simulink model "tester37311"  (R2022b)
settings: Solver=VariableStepAuto  StartTime=0.0  StopTime=25  RelTol=1e-3
values from neighbouring files (symbols this model uses):
  IPR = 0.99    [dane.m]    (also in tester23.m; wykresownik33.m; wykresownik35.m; wykresownik36.m)
  Ng_safe = 1.25    [dane.m]    (also in tester23.m; wykresownik33.m; wykresownik35.m; wykresownik36.m)
  Np = linspace(0.5,2,101)    [dane.m]    (also in tester23.m; untitled.m = 2303; wykresownik33.m; wykresownik35.m)
  Np_safe = 1.25    [dane.m]    (also in tester23.m; wykresownik33.m; wykresownik35.m; wykresownik36.m)
  optimal_rotation = 11.8694    [dane.m]    (also in wykresownik37311.m; wykresownikfinalny.m)
  P3tDIVP2t_perf = 1.0101    [dane.m]    (also in tester23.m = 1; wykresownik33.m = 1; wykresownik35.m = 1; wykresownik36.m = 1)
  P3tDIVP2t_safe = 1.35    [dane.m]    (also in tester23.m; wykresownik33.m; wykresownik35.m; wykresownik36.m)
  Q = 1./Np    [dane.m]    (also in tester23.m; wykresownik33.m; wykresownik35.m; wykresownik36.m)
  Q_safe = 1.15    [dane.m]    (also in tester23.m; wykresownik33.m; wykresownik35.m; wykresownik36.m)
  T45_perf = 1    [dane.m]    (also in tester23.m; wykresownik33.m; wykresownik35.m; wykresownik36.m)
  T45_safe = 1.3    [dane.m]    (also in tester23.m; wykresownik33.m; wykresownik35.m; wykresownik36.m)
  Wf = max(min((1-xfuel)*44,55),33)/1000    [dane.m]    (also in wykresownik37311.m; wykresownikfinalny.m = max(min((1-xfuel)*44,55),33)/100)
  xfuel = linspace(-1,1,201)    [dane.m]    (also in wykresownik37311.m; wykresownikfinalny.m)
libraries: fl_lib x5, sh_lib x4, nesl_utility x4, slpidlib x2, simulink x1
settings Model: Creator=48519  LastModifiedBy=48519
settings ModelReferenceCC: EnableRefExpFcnMdlSchedulingChecks=on

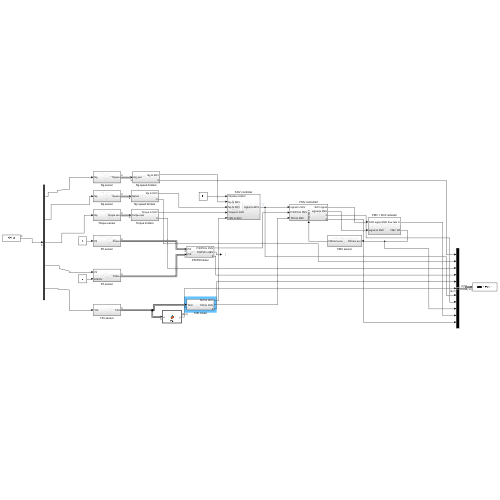
[thumbnail: Simulink's stored preview of the top-level diagram]
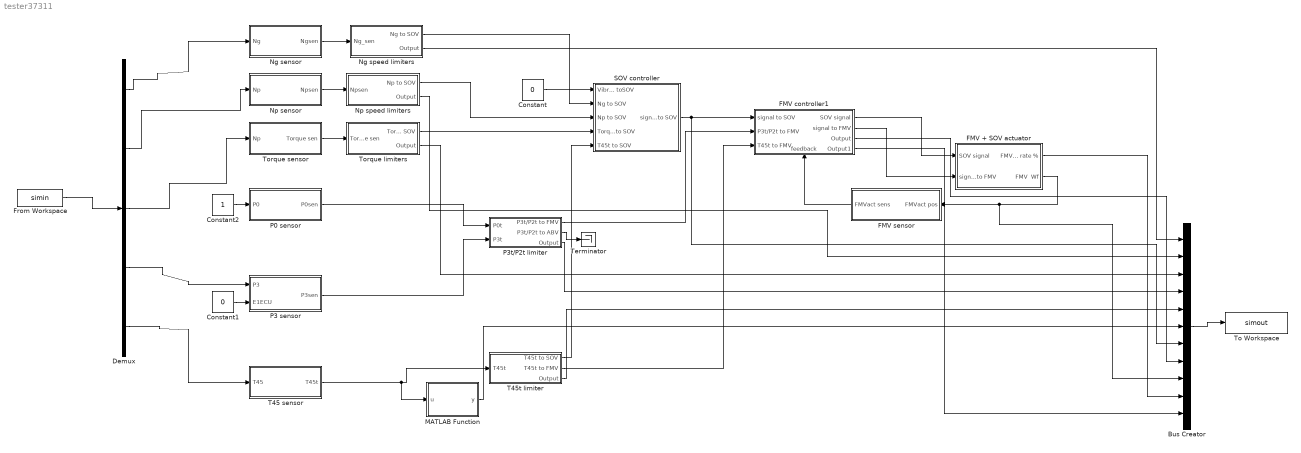
== system tester37311 ==
  " FMV controller1" : Subsystem
      settings: PortSchema="{\"entries\":[{\"content\":{\"sides\":[{\"content\":{\"connectorIds\":[\"In1\",\"In2\",\"In3\"]},\"type\":\"ConnectorPlacement.EquallySpacedRectSide\",\"uuid\":\"38a2bfe9-8c47-42f1-bcd8-9832b9b327c4\"},{\"content\":{\"connectorIds\":[\"Out1\",\"Out2\",\"Out3\",\"Out4\"],\"side\":\"RIGHT\"},\"type\":\"ConnectorPlacement.EquallySpacedRectSide\",\"uuid\":\"0c090e16-2748-47be-b0e4-e5bed405b7d9\"},{\"content\":{\"connectorIds\":[],\"side\":\"TOP\"},\"type\":\"ConnectorPlacement.EquallySpacedRectSide\",\"uuid\":\"289f8d23-a454-4bfb-b029-d000a7415460\"},{\"content\":{\"connectorIds\":[\"In4\"],\"side\":\"BOTTOM\"},\"type\":\"ConnectorPlacement.EquallySpacedRectSide\",\"uuid\":\"f8021000-ba0a-47f6-928e-a2ead77e7ac1\"}]},\"type\":\"ConnectorPlacement.EquallySpacedConnector\",\"uuid\":\"1bac82f5-ade2-4038-9fa3-c74e21ed34d4\"}],\"packageUris\":[\"http://schema.mathworks.com/mf0/Connector/R2020b\"],\"version\":\"1.0\"}"
  Bus Creator : BusCreator  Inputs=11
  Constant : Constant  Value=0
  Constant1 : Constant  Value=0
  Constant2 : Constant
  Demux : Demux  Outputs=5
  FMV + SOV actuator : Subsystem
  FMV sensor : Subsystem
  From Workspace : FromWorkspace  VariableName=simin
  MATLAB Function : MATLAB Function  TreatAsAtomicUnit=on
  Ng sensor : Subsystem
  Ng speed limiters : Subsystem
  Np sensor : Subsystem
  Np speed limiters : Subsystem
  P0 sensor : Subsystem
  P3 sensor : Subsystem
  P3t/P2t limiter : Subsystem
  SOV controller : Subsystem
  T45 sensor : Subsystem
  T45t limiter : Subsystem
  Terminator : Terminator
  To Workspace : ToWorkspace  VariableName=simout  SaveFormat=Timeseries  SampleTime=-1
  Torque limiters : Subsystem
  Torque sensor : Subsystem
  wires:
  P0 sensor/1(P0sen) -> P3t/P2t limiter/1(P0t)
  P3 sensor/1(P3sen) -> P3t/P2t limiter/2(P3t)
  T45 sensor/1(T45t) -> MATLAB Function/1(u), T45t limiter/1(T45t)
  T45t limiter/2(T45t to FMV) -> " FMV controller1"/3(T45t to FMV)
  " FMV controller1"/1(SOV signal) -> FMV + SOV actuator/1(SOV signal)
  " FMV controller1"/2(signal to FMV) -> FMV + SOV actuator/2(signal to FMV)
  FMV sensor/1(FMVact sens) -> " FMV controller1"/4(feedback)
  FMV + SOV actuator/2(FMV  Wf) -> Bus Creator/9, FMV sensor/1(FMVact pos)
  P3t/P2t limiter/1(P3t/P2t to FMV) -> " FMV controller1"/2(P3t/P2t to FMV)
  P3t/P2t limiter/2(P3t/P2t to ABV) -> Terminator/1
  Constant/1 -> SOV controller/1(Vibration toSOV)
  Constant1/1 -> P3 sensor/2(E1ECU)
  Torque sensor/1(Torque sen) -> Torque limiters/1(Torque sen)
  Np sensor/1(Npsen) -> Np speed limiters/1(Npsen)
  Ng sensor/1(Ngsen) -> Ng speed limiters/1(Ng_sen)
  Torque limiters/1(Torque to SOV) -> SOV controller/4(Torque to SOV)
  Np speed limiters/1(Np to SOV) -> SOV controller/3(Np to SOV)
  Ng speed limiters/1(Ng to SOV) -> SOV controller/2(Ng to SOV)
  From Workspace/1 -> Demux/1
  Demux/5 -> T45 sensor/1(T45)
  Demux/4 -> P3 sensor/1(P3)
  Demux/1 -> Ng sensor/1(Ng)
  T45t limiter/1(T45t to SOV) -> SOV controller/5(T45t to SOV)
  Demux/2 -> Np sensor/1(Np)
  Demux/3 -> Torque sensor/1(Np)
  Ng speed limiters/2(Output) -> Bus Creator/1
  P3t/P2t limiter/3(Output) -> Bus Creator/4
  T45t limiter/3(Output) -> Bus Creator/5
  SOV controller/1(signal to SOV) -> Bus Creator/7, " FMV controller1"/1(signal to SOV)
  Np speed limiters/2(Output) -> Bus Creator/2
  Torque limiters/2(Output) -> Bus Creator/3
  Constant2/1 -> P0 sensor/1(P0)
  MATLAB Function/1(y) -> Bus Creator/6
  Bus Creator/1 -> To Workspace/1
  FMV + SOV actuator/1(FMV flow rate %) -> Bus Creator/10
  " FMV controller1"/3(Output) -> Bus Creator/8
  " FMV controller1"/4(Output1) -> Bus Creator/11

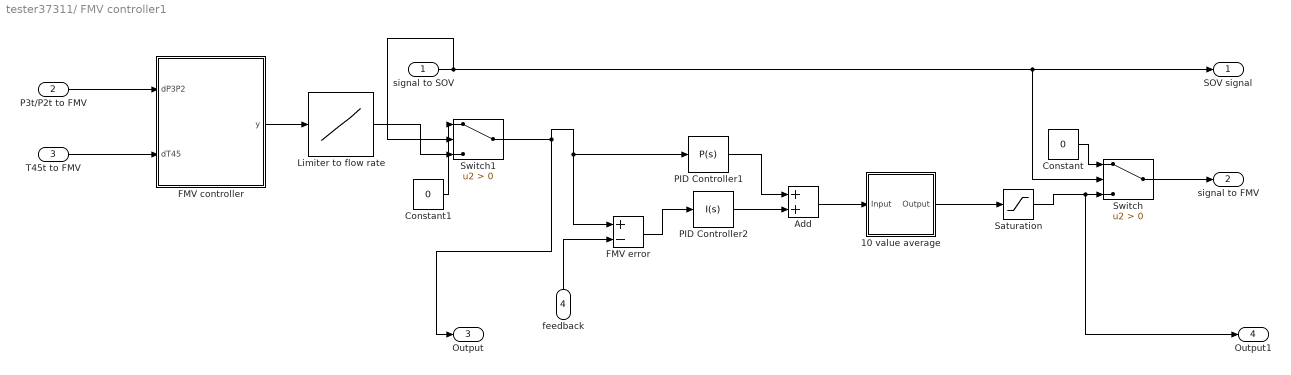
== system tester37311/ FMV controller1 ==
  signal to SOV : Inport
  P3t/P2t to FMV : Inport  Port=2
  T45t to FMV : Inport  Port=3
  feedback : Inport  Port=4
  10 value average : Subsystem
  Add : Sum
  Constant : Constant  Value=0
  Constant1 : Constant  Value=0
  FMV controller : MATLAB Function  TreatAsAtomicUnit=on
  FMV error : Sum  Inputs=+-
  Limiter to flow rate : Lookup_n-D  NumberOfTableDimensions=1  BreakpointsForDimension1=xfuel  Table=Wf  InternalRulePriority=Speed  RndMeth=Simplest
  PID Controller1 : slpidlib/PID Controller  Controller=P  Form=Parallel  TimeDomain=Continuous-time  UseExternalTs=off  SampleTime=-1  IntegratorMethod=Forward Euler  FilterMethod=Forward Euler  ControllerParametersSource=internal  P=11.8694/0.044  I=0  UseKiTs=off  D=0  N=100  UseFilter=on  TunerSelectOption=Transfer Function Based (PID Tuner App)  InitialConditionSource=internal  InitialConditionForIntegrator=0  InitialConditionForFilter=0  DifferentiatorICPrevScaledInput=0  ExternalReset=none  TrackingMode=off  Kt=1  LimitOutput=off  SatLimitsSource=internal  UpperSaturationLimit=inf  LowerSaturationLimit=-inf  LinearizeAsGain=on  AntiWindupMode=none  Kb=1  LimitIntegrator=off  UpperIntegratorSaturationLimit=inf  LowerIntegratorSaturationLimit=-inf  POutMin=[]  POutMax=[]  IOutMin=[]  IOutMax=[]  DOutMin=[]  DOutMax=[]  NOutMin=[]  NOutMax=[]  SumOutMin=[]  SumOutMax=[]  SaturationOutMin=[]  SaturationOutMax=[]  PParamMin=[]  PParamMax=[]  IParamMin=[]  IParamMax=[]  DParamMin=[]  DParamMax=[]  NParamMin=[]  NParamMax=[]  KbParamMin=[]  KbParamMax=[]  KtParamMin=[]  KtParamMax=[]  KbOutMin=[]  KbOutMax=[]  KtOutMin=[]  KtOutMax=[]  IntegratorOutMin=[]  IntegratorOutMax=[]  FilterOutMin=[]  FilterOutMax=[]  SumI1OutMin=[]  SumI1OutMax=[]  SumI2OutMin=[]  SumI2OutMax=[]  SumI3OutMin=[]  SumI3OutMax=[]  SumI4OutMin=[]  SumI4OutMax=[]  SumDOutMin=[]  SumDOutMax=[]  DifferentiatorOutMin=[]  DifferentiatorOutMax=[]  FilterDiffOutCoefMin=[]  FilterDiffOutCoefMax=[]  ReciprocalOutMin=[]  ReciprocalOutMax=[]  SumDenOutMin=[]  SumDenOutMax=[]  SumNumOutMin=[]  SumNumOutMax=[]  DivideOutMin=[]  DivideOutMax=[]  UdiffTsProdOutMin=[]  UdiffTsProdOutMax=[]  NTsProdOutMin=[]  NTsProdOutMax=[]  UintegralTsProdOutMin=[]  UintegralTsProdOutMax=[]  UngainTsProdOutMin=[]  UngainTsProdOutMax=[]  ClampingZeroOutDataTypeStr=Inherit: Inherit via back propagation  ClampingZeroOutMin=[]  ClampingZeroOutMax=[]  FilterDenConstantOutDataTypeStr=Inherit: Inherit via back propagation  FilterDenConstantOutMin=[]  FilterDenConstantOutMax=[]  PCopyOutDataTypeStr=Inherit: Inherit via back propagation  PCopyOutMin=[]  PCopyOutMax=[]  NCopyOutDataTypeStr=Inherit: Inherit via back propagation  NCopyOutMin=[]  NCopyOutMax=[]  IntegratorContinuousStateAttributes=''  IntegratorStateMustResolveToSignalObject=off  IntegratorRTWStateStorageClass=Auto  FilterContinuousStateAttributes=''  FilterStateMustResolveToSignalObject=off  FilterRTWStateStorageClass=Auto  ParallelPVariant=InternalParameters  IdealPVariant=Disabled  IVariant=Disabled  DVariant=Disabled  IntegratorVariant=Disabled  SatVariant=Disabled  AWVariant=Disabled  PCopyVariant=Disabled  TRVariant=Disabled  FdbkBlocksVariant=Forward  IdealPFdbkVariant=Disabled  SatFdbkVariant=Disabled  DerivativeFilterVariant=Disabled  NVariant=Disabled  NCopyVariant=Disabled_SignalSpec  FilterICVariant=Disabled  IntegratorICVariant=Disabled  ExternalResetVariant=Disabled  TRSumVariant=Passthrough  SumFdbkVariant=Disabled  SumVariant=Passthrough_P  TsampFilterVariant=InternalTs  TsampNgainVariant=Passthrough  TsampIntegralVariant=Disabled_SignalSpec  ExternalSaturationOutDataTypeStr=Inherit: Same as second input
  PID Controller2 : slpidlib/PID Controller  Controller=I  Form=Parallel  TimeDomain=Continuous-time  UseExternalTs=off  SampleTime=-1  IntegratorMethod=Forward Euler  FilterMethod=Forward Euler  ControllerParametersSource=internal  P=1  I=0.01  UseKiTs=off  D=0  N=100  UseFilter=on  TunerSelectOption=Transfer Function Based (PID Tuner App)  InitialConditionSource=internal  InitialConditionForIntegrator=0  InitialConditionForFilter=0  DifferentiatorICPrevScaledInput=0  ExternalReset=none  TrackingMode=off  Kt=1  LimitOutput=on  SatLimitsSource=internal  UpperSaturationLimit=inf  LowerSaturationLimit=-inf  LinearizeAsGain=on  AntiWindupMode=clamping  Kb=1  LimitIntegrator=on  UpperIntegratorSaturationLimit=10  LowerIntegratorSaturationLimit=-10  POutMin=[]  POutMax=[]  IOutMin=[]  IOutMax=[]  DOutMin=[]  DOutMax=[]  NOutMin=[]  NOutMax=[]  SumOutMin=[]  SumOutMax=[]  SaturationOutMin=[]  SaturationOutMax=[]  PParamMin=[]  PParamMax=[]  IParamMin=[]  IParamMax=[]  DParamMin=[]  DParamMax=[]  NParamMin=[]  NParamMax=[]  KbParamMin=[]  KbParamMax=[]  KtParamMin=[]  KtParamMax=[]  KbOutMin=[]  KbOutMax=[]  KtOutMin=[]  KtOutMax=[]  IntegratorOutMin=[]  IntegratorOutMax=[]  FilterOutMin=[]  FilterOutMax=[]  SumI1OutMin=[]  SumI1OutMax=[]  SumI2OutMin=[]  SumI2OutMax=[]  SumI3OutMin=[]  SumI3OutMax=[]  SumI4OutMin=[]  SumI4OutMax=[]  SumDOutMin=[]  SumDOutMax=[]  DifferentiatorOutMin=[]  DifferentiatorOutMax=[]  FilterDiffOutCoefMin=[]  FilterDiffOutCoefMax=[]  ReciprocalOutMin=[]  ReciprocalOutMax=[]  SumDenOutMin=[]  SumDenOutMax=[]  SumNumOutMin=[]  SumNumOutMax=[]  DivideOutMin=[]  DivideOutMax=[]  UdiffTsProdOutMin=[]  UdiffTsProdOutMax=[]  NTsProdOutMin=[]  NTsProdOutMax=[]  UintegralTsProdOutMin=[]  UintegralTsProdOutMax=[]  UngainTsProdOutMin=[]  UngainTsProdOutMax=[]  ClampingZeroOutDataTypeStr=Inherit: Inherit via back propagation  ClampingZeroOutMin=[]  ClampingZeroOutMax=[]  FilterDenConstantOutDataTypeStr=Inherit: Inherit via back propagation  FilterDenConstantOutMin=[]  FilterDenConstantOutMax=[]  PCopyOutDataTypeStr=Inherit: Inherit via back propagation  PCopyOutMin=[]  PCopyOutMax=[]  NCopyOutDataTypeStr=Inherit: Inherit via back propagation  NCopyOutMin=[]  NCopyOutMax=[]  IntegratorContinuousStateAttributes=''  IntegratorStateMustResolveToSignalObject=off  IntegratorRTWStateStorageClass=Auto  FilterContinuousStateAttributes=''  FilterStateMustResolveToSignalObject=off  FilterRTWStateStorageClass=Auto  ParallelPVariant=Disabled  IdealPVariant=Disabled  IVariant=InternalParameters  DVariant=Disabled  IntegratorVariant=Continuous  SatVariant=Enabled  AWVariant=ContClampingParallel  PCopyVariant=Disabled  TRVariant=Disabled  FdbkBlocksVariant=Forward  IdealPFdbkVariant=Disabled  SatFdbkVariant=Disabled  DerivativeFilterVariant=Disabled  NVariant=Disabled  NCopyVariant=Disabled_SignalSpec  FilterICVariant=Disabled  IntegratorICVariant=InternalICs  ExternalResetVariant=Disabled  TRSumVariant=Passthrough  SumFdbkVariant=Disabled  SumVariant=Passthrough_I  TsampFilterVariant=InternalTs  TsampNgainVariant=Passthrough  TsampIntegralVariant=Passthrough  ExternalSaturationOutDataTypeStr=Inherit: Same as second input
  Saturation : Saturate  UpperLimit=11.8694*1.25  LowerLimit=11.8694*0.75
  Switch : Switch  Criteria=u2 > Threshold  SaturateOnIntegerOverflow=off  InputSameDT=off
  Switch1 : Switch  Criteria=u2 > Threshold  SaturateOnIntegerOverflow=off  InputSameDT=off
  SOV signal : Outport
  signal to FMV : Outport  Port=2
  Output : Outport  Port=3
  Output1 : Outport  Port=4
  wires:
  Switch1/1 -> Output/1, PID Controller1/1, FMV error/1
  P3t/P2t to FMV/1 -> FMV controller/1(dP3P2)
  T45t to FMV/1 -> FMV controller/2(dT45)
  FMV controller/1(y) -> Limiter to flow rate/1
  Switch/1 -> signal to FMV/1
  Constant/1 -> Switch/1
  FMV error/1 -> PID Controller2/1
  PID Controller1/1 -> Add/1
  PID Controller2/1 -> Add/2
  Add/1 -> 10 value average/1(Input)
  Saturation/1 -> Output1/1, Switch/3
  signal to SOV/1 -> Switch1/2, Switch/2, SOV signal/1
  feedback/1 -> FMV error/2
  10 value average/1(Output) -> Saturation/1
  Limiter to flow rate/1 -> Switch1/3
  Constant1/1 -> Switch1/1

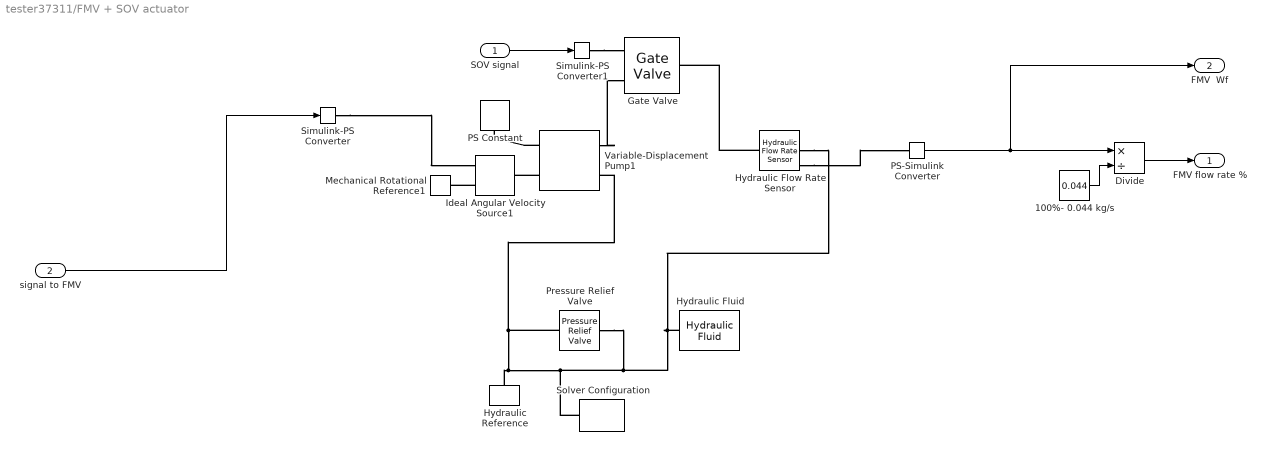
== system tester37311/FMV + SOV actuator ==
  SOV signal : Inport
  signal to FMV : Inport  Port=2
  100%- 0.044 kg/s : Constant  Value=0.044
  Divide : Product  Inputs=*/
  Gate Valve : sh_lib/Valves/Flow Control Valves/Gate Valve  d_gate=0.01 m  x_0=-0.1 m  C_d=10^12  A_leak=1e-12 m^2  lam_spec=1  B_lam=0.999  Re_cr=10
      settings: InternalSimscapePortConfiguration="{\"Bottom\":[],\"Left\":[{\"id\":\"S\",\"label\":\"S\",\"type\":\"input\"},{\"id\":\"A\",\"label\":\"A\",\"type\":\"foundation.hydraulic.hydraulic\"}],\"Right\":[{\"id\":\"B\",\"label\":\"B\",\"type\":\"foundation.hydraulic.hydraulic\"}],\"Top\":[]}"
  Hydraulic Flow Rate Sensor : fl_lib/Hydraulic/Hydraulic Sensors/Hydraulic Flow Rate Sensor
  Hydraulic Fluid : sh_lib/Hydraulic Utilities/Hydraulic Fluid  SelFluid=22  SysTemp=60  TrapAir=0.005  ViscDerFactor=1  range_error=2
  Hydraulic Reference : fl_lib/Hydraulic/Hydraulic Elements/Hydraulic Reference
  Ideal Angular Velocity Source1 : fl_lib/Mechanical/Mechanical Sources/Ideal Angular Velocity Source
  Mechanical Rotational Reference1 : fl_lib/Mechanical/Rotational Elements/Mechanical Rotational Reference
  PS Constant : fl_lib/Physical Signals/Sources/PS Constant  constant=1
  PS-Simulink Converter : nesl_utility/PS-Simulink Converter  PhysicalDomain=network_engine_domain  SubClassName=ps_output  LeftPortType=input  RightPortType=output  PseudoPeriodic=off  Frequencies=[]  VectorFormat=inherit  Unit=inherit  AffineConversion=off
  Pressure Relief Valve : sh_lib/Valves/Pressure Control Valves/Pressure Relief Valve  valve_area_spec=1  p_diff_TLU=[30.15e5 : 15e3 : 31.35e5] Pa  area_TLU=[1 : 1 : 9] .* 1e-5 m^2  area_max=1e-4 m^2  pres_set=50e5 Pa  reg_range=5e5 Pa  C_d=0.7  A_leak=1e-12 m^2  lam_spec=1  B_lam=0.999  Re_cr=12  dynamic=0  tau=0.1 s  area_init=1e-12 m^2
      settings: InternalSimscapePortConfiguration="{\"Bottom\":[],\"Left\":[{\"id\":\"A\",\"label\":\"A\",\"type\":\"foundation.hydraulic.hydraulic\"}],\"Right\":[{\"id\":\"B\",\"label\":\"B\",\"type\":\"foundation.hydraulic.hydraulic\"}],\"Top\":[]}"
  Simulink-PS Converter : nesl_utility/Simulink-PS Converter  PhysicalDomain=network_engine_domain  SubClassName=ps_input  LeftPortType=input  RightPortType=output  PseudoPeriodic=off  Frequencies=[]  NoiseDistribution=none  NoiseParameters=[]  Unit=1  AffineConversion=off  FilteringAndDerivatives=provide  SimscapeFilterOrder=1  InputFilterTimeConstant=0.001  UdotUserProvided=0
  Simulink-PS Converter1 : nesl_utility/Simulink-PS Converter  PhysicalDomain=network_engine_domain  SubClassName=ps_input  LeftPortType=input  RightPortType=output  PseudoPeriodic=off  Frequencies=[]  NoiseDistribution=none  NoiseParameters=[]  Unit=1  AffineConversion=off  FilteringAndDerivatives=provide  SimscapeFilterOrder=1  InputFilterTimeConstant=0.001  UdotUserProvided=0
  Solver Configuration : nesl_utility/Solver Configuration  PhysicalDomain=network_engine_domain  SubClassName=solver  LeftPortType=input  RightPortType=generic  Tones=[]  Harmonics=[]  SimulateNoise=off  Profile=off  UseLocalSampling=off  EnableSwitchedLinearOptims=on  FrequencyDomain=off  UseCCode=off  RelTol=0.001  AbsTol=0.001  MinStep=1e-09  ToWorkspace=off  RevertToSquareIcSolve=off  NumHomotopyIterations=100  PhasorMode=off  PhasorModeNumHarmonics=1  ConsistencySolver=NEWTON_XTOL_AFTER_FTOL  IndexReductionMethod=DerivativeReplacement  DoDC=off  ResidualTolerance=1e-09  ConsistencyTolSource=GLOBAL  ConsistencyAbsTol=0.001  ConsistencyRelTol=0.001  ConsistencyTolFactor=0.001  UseLocalSolver=off  LocalSolverChoice=NE_BACKWARD_EULER_ADVANCER  ResolveIndetEquations=on  FunctionEvalNumThread=1  LocalSolverSampleTime=0.001  DoFixedCost=off  MaxNonlinIter=3  MaxModeIter=2  ComputeImpulses=off  ImpulseIterations=2  LinearAlgebra=auto  LinearAlgebraNumThread=0  EquationFormulation=NE_TIME_EF  DelaysMemoryBudget=1024  AutomaticFiltering=on  FilteringTimeConstant=0.001  PartitionStorageMethod=AS_NEEDED  PartitionMemoryBudget=1024  PartitionMethod=ROBUST
  Variable-Displacement Pump1 : sh_lib/Pumps and Motors/Variable-Displacement Pump  mdl_type=1  stroke_max=0.005 m  D_max=30 cm^3/rev  cntrl_mem_tab=[-.0075, -.0025, 0, .0025, .0075] m  displ_tab=[-30, -19, 0, 19, 30] cm^3/rev  interp_method=1  extrap_method=1  loss_spec=1  w_nominal=188 rad/s  pr_nominal=100e5 Pa  visc_nominal=18 cSt  dens_nominal=900 kg/m^3  efficiency_vol=0.92  no_load_torque=0.05 N*m  torque_pressure_coeff=0.6e-6 N*m/Pa  p_diff_eff_TLU=[100000, 1000000, 2000000] Pa  omega_eff_TLU=[25, 50, 100, 200, 300, 400] rad/s  displacement_eff_TLU=[-30, -19, 19, 30] cm^3/rev  vol_eff_TLU=repmat([.816, .908, .954, .977, .981, .984; .325, .663, .831, .916, .925, .946; .137, .568, .78, .892, .893, .91], 1, 1, 4)  mech_eff_TLU=repmat([.996, .996, .996, .996, .996, .996; .988, .989, .989, .989, .989, .99; .981, .981, .982, .982, .983, .984], 1, 1, 4)  p_diff_loss_TLU=[100000, 1000000, 2000000] Pa  omega_loss_TLU=[25, 50, 100, 200, 300, 400] rad/s  displacement_loss_TLU=[-30, -19, 19, 30] cm^3/rev  vol_loss_TLU=repmat([.023, .023, .023, .023, .0285, .032; .0844, .0842, .0845, .084, .1125, .108; .1079, .108, .11, .108, .1605, .18] * 1e-3, 1, 1, 4) m^3/s  mech_loss_TLU=repmat([.002, .002, .002, .002, .002, .002; .0607, .0556, .0556, .0556, .0556, .0505; .1937, .1937, .1833, .1833, .1729, .1626], 1, 1, 4) N*m  pressure_threshold=1e5 Pa  omega_threshold=10 rad/s  displacement_threshold=0.5 cm^3/rev  octant_check=0  pressure_check=0  min_valid_pressure=0 Pa  vol_eff_min=1e-3  vol_eff_max=1  mech_eff_min=1e-3  mech_eff_max=1
      settings: InternalSimscapePortConfiguration="{\"Bottom\":[],\"Left\":[{\"id\":\"C\",\"label\":\"C\",\"type\":\"input\"},{\"id\":\"S\",\"label\":\"S\",\"type\":\"foundation.mechanical.rotational.rotational\"}],\"Right\":[{\"id\":\"P\",\"label\":\"P\",\"type\":\"foundation.hydraulic.hydraulic\"},{\"id\":\"T\",\"label\":\"T\",\"type\":\"foundation.hydraulic.hydraulic\"}],\"Top\":[]}"
  FMV flow rate % : Outport
  FMV  Wf : Outport  Port=2
  wires:
  PS-Simulink Converter/1 -> FMV  Wf/1, Divide/1
  signal to FMV/1 -> Simulink-PS Converter/1
  100%- 0.044 kg/s/1 -> Divide/2
  Divide/1 -> FMV flow rate %/1
  SOV signal/1 -> Simulink-PS Converter1/1
  connections:
  Pressure Relief Valve/RConn1 -- Hydraulic Flow Rate Sensor/RConn2 -- Hydraulic Fluid/RConn1 -- Variable-Displacement Pump1/RConn2 -- Pressure Relief Valve/LConn1 -- Hydraulic Reference/LConn1 -- Solver Configuration/RConn1
  Simulink-PS Converter/RConn1 -- Ideal Angular Velocity Source1/RConn1
  Ideal Angular Velocity Source1/RConn2 -- Mechanical Rotational Reference1/LConn1
  Variable-Displacement Pump1/LConn2 -- Ideal Angular Velocity Source1/LConn1
  Hydraulic Flow Rate Sensor/RConn3 -- PS-Simulink Converter/LConn1
  Variable-Displacement Pump1/LConn1 -- PS Constant/RConn1
  Simulink-PS Converter1/RConn1 -- Gate Valve/LConn1
  Variable-Displacement Pump1/RConn1 -- Gate Valve/LConn2
  Hydraulic Flow Rate Sensor/LConn1 -- Gate Valve/RConn1

== system tester37311/FMV sensor ==
  FMVact pos : Inport
  Add2 : Sum
  Derivative : Derivative
  Integrator : Integrator  InitialCondition=1
  Product2 : Product
  Rate 100Hz1 : RateTransition  OutPortSampleTimeMultiple=2  OutPortSampleTime=1
  normal noise1 : UniformRandomNumber  Seed=1  SampleTime=0.1
  FMVact sens : Outport
  wires:
  Rate 100Hz1/1 -> Add2/1, Product2/1
  Add2/1 -> Integrator/1
  FMVact pos/1 -> Derivative/1
  normal noise1/1 -> Product2/2
  Product2/1 -> Add2/2
  Derivative/1 -> Rate 100Hz1/1
  Integrator/1 -> FMVact sens/1

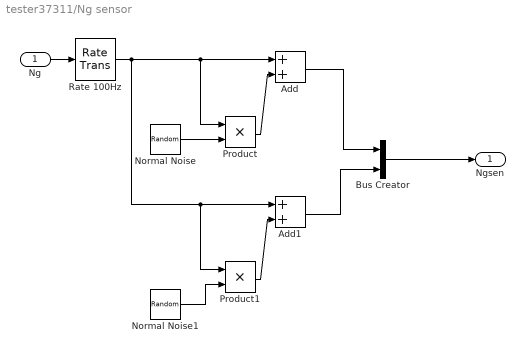
== system tester37311/Ng sensor ==
  Ng : Inport
  Add : Sum
  Add1 : Sum
  Bus Creator : BusCreator  Inputs=2
  Normal Noise : RandomNumber  Variance=((0.017)^2)*pi/2  Seed=10  SampleTime=0.01
  Normal Noise1 : RandomNumber  Variance=((0.017)^2)*pi/2  Seed=11  SampleTime=0.01
  Product : Product
  Product1 : Product
  Rate 100Hz : RateTransition  OutPortSampleTimeMultiple=2  OutPortSampleTime=0.01
  Ngsen : Outport
  wires:
  Product/1 -> Add/2
  Product1/1 -> Add1/2
  Normal Noise1/1 -> Product1/2
  Rate 100Hz/1 -> Add/1, Product/1, Add1/1, Product1/1
  Ng/1 -> Rate 100Hz/1
  Add1/1 -> Bus Creator/2
  Add/1 -> Bus Creator/1
  Bus Creator/1 -> Ngsen/1
  Normal Noise/1 -> Product/2

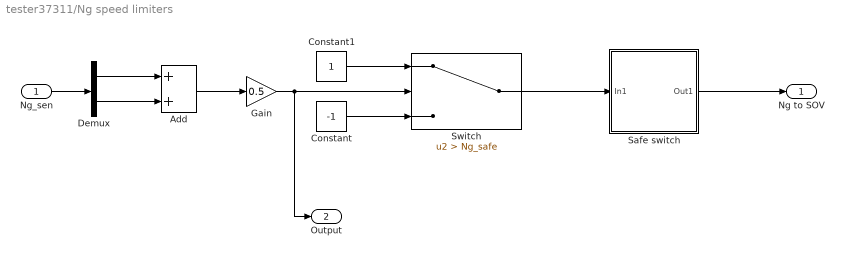
== system tester37311/Ng speed limiters ==
  Ng_sen : Inport
  Add : Sum
  Constant : Constant  Value=-1
  Constant1 : Constant
  Demux : Demux  Outputs=2
  Gain : Gain  Gain=0.5
  Safe switch : Subsystem
  Switch : Switch  Criteria=u2 > Threshold  Threshold=Ng_safe  SaturateOnIntegerOverflow=off  InputSameDT=off
  Ng to SOV : Outport
  Output : Outport  Port=2
  wires:
  Constant/1 -> Switch/3
  Constant1/1 -> Switch/1
  Ng_sen/1 -> Demux/1
  Demux/1 -> Add/1
  Demux/2 -> Add/2
  Gain/1 -> Output/1, Switch/2
  Add/1 -> Gain/1
  Switch/1 -> Safe switch/1(In1)
  Safe switch/1(Out1) -> Ng to SOV/1

== system tester37311/Np sensor ==
  Np : Inport
  Add : Sum
  Add1 : Sum
  Bus Creator : BusCreator  Inputs=2
  Normal Noise1 : RandomNumber  Variance=((0.017)^2)*pi/2  Seed=13  SampleTime=0.01
  Normal Noise2 : RandomNumber  Variance=((0.017)^2)*pi/2  Seed=14  SampleTime=0.01
  Product : Product
  Product1 : Product
  Rate 100Hz : RateTransition  OutPortSampleTimeMultiple=2  OutPortSampleTime=0.01
  Npsen : Outport
  wires:
  Normal Noise1/1 -> Product/2
  Product/1 -> Add/2
  Np/1 -> Rate 100Hz/1
  Normal Noise2/1 -> Product1/2
  Product1/1 -> Add1/2
  Rate 100Hz/1 -> Add/1, Product/1, Add1/1, Product1/1
  Add1/1 -> Bus Creator/2
  Add/1 -> Bus Creator/1
  Bus Creator/1 -> Npsen/1

== system tester37311/Np speed limiters ==
  Npsen : Inport
  Add : Sum
  Constant : Constant  Value=-1
  Constant1 : Constant
  Demux : Demux  Outputs=2
  Gain : Gain  Gain=0.5
  Safe switch : Subsystem
  Switch : Switch  Criteria=u2 > Threshold  Threshold=Np_safe  SaturateOnIntegerOverflow=off  InputSameDT=off
  Np to SOV : Outport
  Output : Outport  Port=2
  wires:
  Switch/1 -> Safe switch/1(In1)
  Constant1/1 -> Switch/1
  Constant/1 -> Switch/3
  Gain/1 -> Output/1, Switch/2
  Demux/2 -> Add/2
  Npsen/1 -> Demux/1
  Add/1 -> Gain/1
  Demux/1 -> Add/1
  Safe switch/1(Np to SOV) -> Np to SOV/1

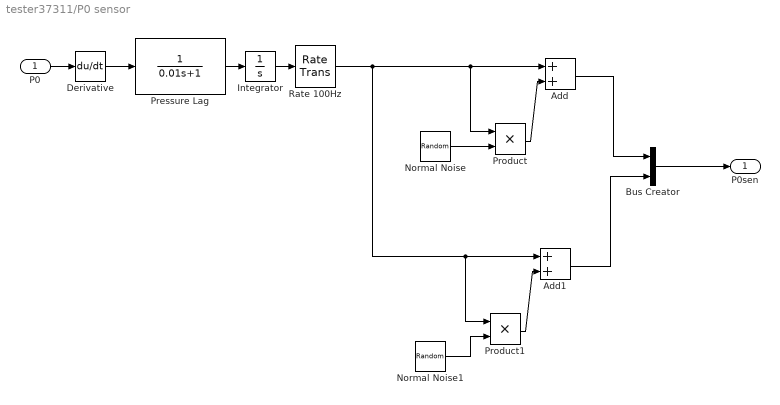
== system tester37311/P0 sensor ==
  P0 : Inport
  Add : Sum
  Add1 : Sum
  Bus Creator : BusCreator  Inputs=2
  Derivative : Derivative
  Integrator : Integrator  InitialCondition=1
  Normal Noise : RandomNumber  Variance=((0.005)^2)*pi/2  Seed=31  SampleTime=0.01
  Normal Noise1 : RandomNumber  Variance=((0.005)^2)*pi/2  Seed=33  SampleTime=0.01
  Pressure Lag : TransferFcn  Denominator=[0.01 1]
  Product : Product
  Product1 : Product
  Rate 100Hz : RateTransition  OutPortSampleTimeMultiple=2  OutPortSampleTime=0.01
  P0sen : Outport
  wires:
  P0/1 -> Derivative/1
  Normal Noise1/1 -> Product1/2
  Normal Noise/1 -> Product/2
  Add1/1 -> Bus Creator/2
  Pressure Lag/1 -> Integrator/1
  Bus Creator/1 -> P0sen/1
  Product1/1 -> Add1/2
  Product/1 -> Add/2
  Rate 100Hz/1 -> Add1/1, Product1/1, Add/1, Product/1
  Add/1 -> Bus Creator/1
  Derivative/1 -> Pressure Lag/1
  Integrator/1 -> Rate 100Hz/1

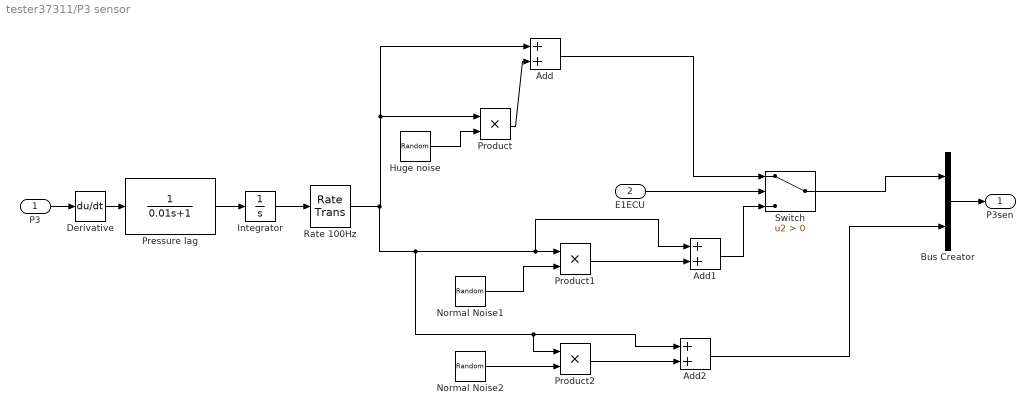
== system tester37311/P3 sensor ==
  P3 : Inport
  E1ECU : Inport  Port=2
  Add : Sum
  Add1 : Sum
  Add2 : Sum
  Bus Creator : BusCreator  Inputs=2
  Derivative : Derivative
  Huge noise : RandomNumber  Variance=((0.03)^2)*pi/2  Seed=1  SampleTime=0.01
  Integrator : Integrator  InitialCondition=1
  Normal Noise1 : RandomNumber  Variance=((0.005)^2)*pi/2  Seed=2  SampleTime=0.01
  Normal Noise2 : RandomNumber  Variance=((0.005)^2)*pi/2  Seed=4  SampleTime=0.01
  Pressure lag : TransferFcn  Numerator=[1 ]  Denominator=[0.01 1]
  Product : Product
  Product1 : Product
  Product2 : Product
  Rate 100Hz : RateTransition  OutPortSampleTimeMultiple=2  OutPortSampleTime=0.01
  Switch : Switch  Criteria=u2 > Threshold  SaturateOnIntegerOverflow=off  InputSameDT=off
  P3sen : Outport
  wires:
  Bus Creator/1 -> P3sen/1
  P3/1 -> Derivative/1
  Normal Noise2/1 -> Product2/2
  Add/1 -> Switch/1
  Huge noise/1 -> Product/2
  Add1/1 -> Switch/3
  Product/1 -> Add/2
  Product2/1 -> Add2/2
  Rate 100Hz/1 -> Add2/1, Product2/1, Add1/1, Product1/1, Product/1, Add/1
  Add2/1 -> Bus Creator/2
  Normal Noise1/1 -> Product1/2
  Switch/1 -> Bus Creator/1
  Pressure lag/1 -> Integrator/1
  E1ECU/1 -> Switch/2
  Product1/1 -> Add1/2
  Derivative/1 -> Pressure lag/1
  Integrator/1 -> Rate 100Hz/1

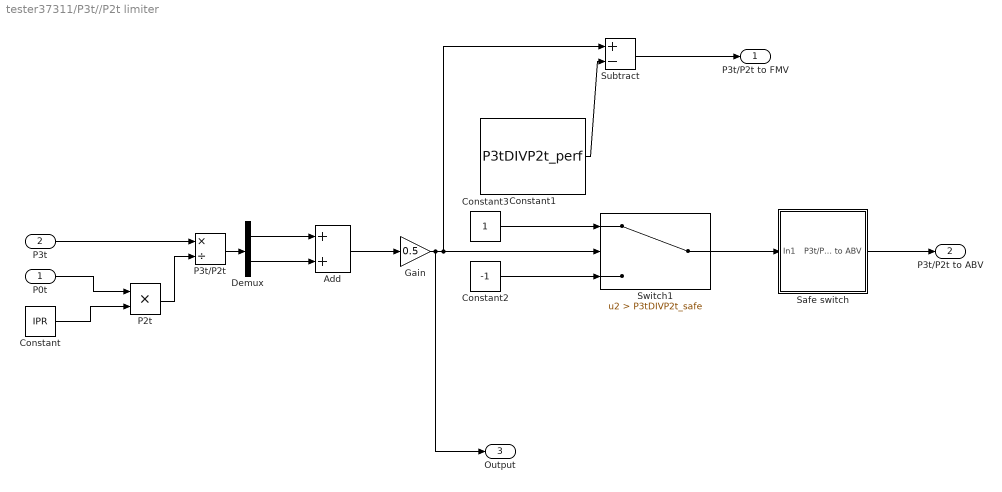
== system tester37311/P3t//P2t limiter ==
  P0t : Inport
  P3t : Inport  Port=2
  Add : Sum
  Constant : Constant  Value=IPR
  Constant1 : Constant  Value=P3tDIVP2t_perf
  Constant2 : Constant  Value=-1
  Constant3 : Constant
  Demux : Demux  Outputs=2
  Gain : Gain  Gain=0.5
  P2t : Product
  P3t/P2t : Product  Inputs=*/
  Safe switch : Subsystem
  Subtract : Sum  Inputs=+-
  Switch1 : Switch  Criteria=u2 > Threshold  Threshold=P3tDIVP2t_safe  SaturateOnIntegerOverflow=off  InputSameDT=off
  P3t/P2t to FMV : Outport
  P3t/P2t to ABV : Outport  Port=2
  Output : Outport  Port=3
  wires:
  Subtract/1 -> P3t/P2t to FMV/1
  P3t/1 -> P3t/P2t/1
  Constant1/1 -> Subtract/2
  Gain/1 -> Output/1, Switch1/2, Subtract/1
  Constant2/1 -> Switch1/3
  Switch1/1 -> Safe switch/1(In1)
  Constant3/1 -> Switch1/1
  Demux/2 -> Add/2
  Demux/1 -> Add/1
  Add/1 -> Gain/1
  P3t/P2t/1 -> Demux/1
  Safe switch/1(P3t/P2t to ABV) -> P3t/P2t to ABV/1
  P0t/1 -> P2t/1
  P2t/1 -> P3t/P2t/2
  Constant/1 -> P2t/2

== system tester37311/SOV controller ==
  Vibration toSOV : Inport
  Ng to SOV : Inport  Port=2
  Np to SOV : Inport  Port=3
  Torque to SOV : Inport  Port=4
  T45t to SOV : Inport  Port=5
  Add : Sum  Inputs=+++++  OutMax=[1]
  Latch max value : simulink/Math Operations/MinMax Running Resettable  Function=max  vinit=0.0
  NOT RESET : Constant  Value=0
  max=1 : Saturate  UpperLimit=1  LowerLimit=0
  signal to SOV : Outport
  wires:
  Vibration toSOV/1 -> Add/1
  Ng to SOV/1 -> Add/2
  Np to SOV/1 -> Add/3
  T45t to SOV/1 -> Add/4
  Torque to SOV/1 -> Add/5
  NOT RESET/1 -> Latch max value/2
  max=1/1 -> Latch max value/1
  Add/1 -> max=1/1
  Latch max value/1 -> signal to SOV/1

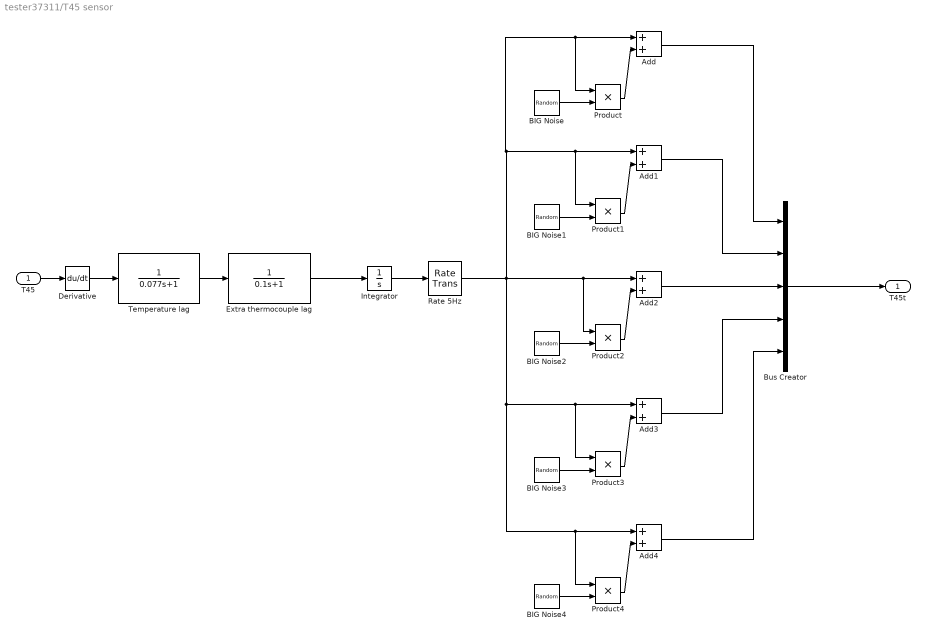
== system tester37311/T45 sensor ==
  T45 : Inport
  Add{,1..4} (5 alike) : Sum
  BIG Noise : RandomNumber  Variance=((0.015)^2)*pi/2  Seed=51  SampleTime=0.2
  BIG Noise1 : RandomNumber  Variance=((0.015)^2)*pi/2  Seed=53  SampleTime=0.2
  BIG Noise2 : RandomNumber  Variance=((0.015)^2)*pi/2  Seed=55  SampleTime=0.2
  BIG Noise3 : RandomNumber  Variance=((0.015)^2)*pi/2  Seed=57  SampleTime=0.2
  BIG Noise4 : RandomNumber  Variance=((0.015)^2)*pi/2  Seed=59  SampleTime=0.2
  Bus Creator : BusCreator  Inputs=5
  Derivative : Derivative
  Extra thermocouple lag : TransferFcn  Denominator=[0.1 1]
  Integrator : Integrator  InitialCondition=1
  Product{,1..4} (5 alike) : Product
  Rate 5Hz : RateTransition  OutPortSampleTime=0.2
  Temperature lag : TransferFcn  Denominator=[0.077 1]
  T45t : Outport
  wires:
  T45/1 -> Derivative/1
  Extra thermocouple lag/1 -> Integrator/1
  Temperature lag/1 -> Extra thermocouple lag/1
  BIG Noise/1 -> Product/2
  Product/1 -> Add/2
  Product1/1 -> Add1/2
  BIG Noise1/1 -> Product1/2
  Product2/1 -> Add2/2
  BIG Noise2/1 -> Product2/2
  Product3/1 -> Add3/2
  BIG Noise3/1 -> Product3/2
  Product4/1 -> Add4/2
  Rate 5Hz/1 -> Add/1, Product/1, Add1/1, Product1/1, Product2/1, Add2/1, Add3/1, Product3/1, Add4/1, Product4/1
  BIG Noise4/1 -> Product4/2
  Bus Creator/1 -> T45t/1
  Add2/1 -> Bus Creator/3
  Add3/1 -> Bus Creator/4
  Add4/1 -> Bus Creator/5
  Add1/1 -> Bus Creator/2
  Add/1 -> Bus Creator/1
  Integrator/1 -> Rate 5Hz/1
  Derivative/1 -> Temperature lag/1

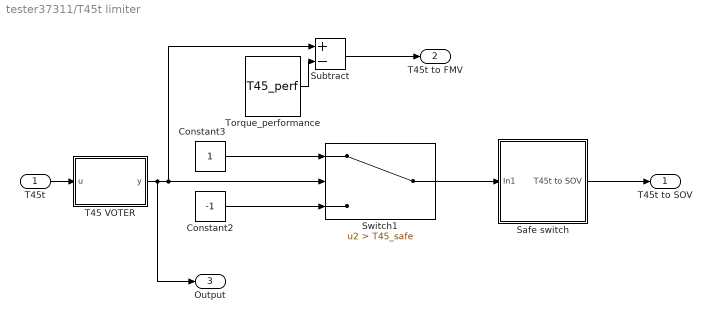
== system tester37311/T45t limiter ==
  T45t : Inport
  Constant2 : Constant  Value=-1
  Constant3 : Constant
  Safe switch : Subsystem
  Subtract : Sum  Inputs=+-
  Switch1 : Switch  Criteria=u2 > Threshold  Threshold=T45_safe  SaturateOnIntegerOverflow=off  InputSameDT=off
  T45 VOTER : MATLAB Function  TreatAsAtomicUnit=on
  Torque_performance : Constant  Value=T45_perf
  T45t to SOV : Outport
  T45t to FMV : Outport  Port=2
  Output : Outport  Port=3
  wires:
  Subtract/1 -> T45t to FMV/1
  ? -> ?
  Switch1/1 -> Safe switch/1(In1)
  Constant2/1 -> Switch1/3
  Constant3/1 -> Switch1/1
  Torque_performance/1 -> Subtract/2
  T45 VOTER/1(y) -> Output/1, Subtract/1, Switch1/2
  T45t/1 -> T45 VOTER/1(u)
  Safe switch/1(T45t to SOV) -> T45t to SOV/1

== system tester37311/Torque limiters ==
  Torque sen : Inport
  Add : Sum
  Constant : Constant  Value=-1
  Constant1 : Constant
  Demux : Demux  Outputs=2
  Gain : Gain  Gain=0.5
  Safe switch : Subsystem
  Switch : Switch  Criteria=u2 > Threshold  Threshold=Q_safe  SaturateOnIntegerOverflow=off  InputSameDT=off
  Torque to SOV : Outport
  Output : Outport  Port=2
  wires:
  Gain/1 -> Output/1, Switch/2
  Constant1/1 -> Switch/1
  Torque sen/1 -> Demux/1
  Constant/1 -> Switch/3
  Demux/2 -> Add/2
  Add/1 -> Gain/1
  Demux/1 -> Add/1
  Switch/1 -> Safe switch/1(In1)
  Safe switch/1(Torque to SOV) -> Torque to SOV/1

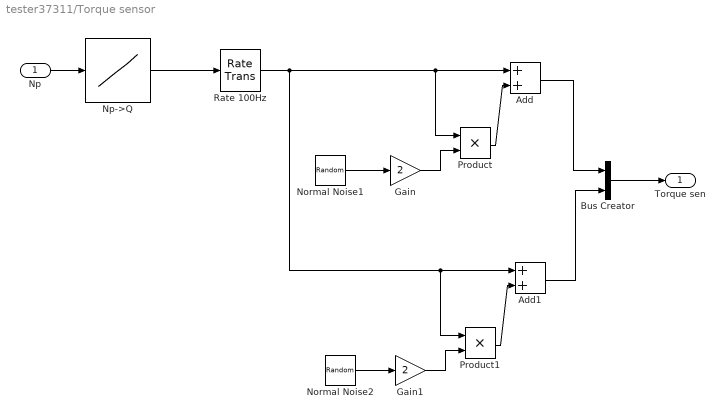
== system tester37311/Torque sensor ==
  Np : Inport
  Add : Sum
  Add1 : Sum
  Bus Creator : BusCreator  Inputs=2
  Gain : Gain  Gain=2
  Gain1 : Gain  Gain=2
  Normal Noise1 : RandomNumber  Variance=((0.017)^2)*pi/2  Seed=21  SampleTime=0.01
  Normal Noise2 : RandomNumber  Variance=((0.017)^2)*pi/2  Seed=23  SampleTime=0.01
  Np->Q : Lookup_n-D  NumberOfTableDimensions=1  BreakpointsForDimension1=Np  Table=Q  InternalRulePriority=Speed  RndMeth=Simplest
  Product : Product
  Product1 : Product
  Rate 100Hz : RateTransition  OutPortSampleTimeMultiple=2  OutPortSampleTime=0.01
  Torque sen : Outport
  wires:
  Normal Noise1/1 -> Gain/1
  Product/1 -> Add/2
  Gain/1 -> Product/2
  Normal Noise2/1 -> Gain1/1
  Product1/1 -> Add1/2
  Gain1/1 -> Product1/2
  Rate 100Hz/1 -> Add1/1, Product1/1, Add/1, Product/1
  Add1/1 -> Bus Creator/2
  Np/1 -> Np->Q/1
  Add/1 -> Bus Creator/1
  Bus Creator/1 -> Torque sen/1
  Np->Q/1 -> Rate 100Hz/1

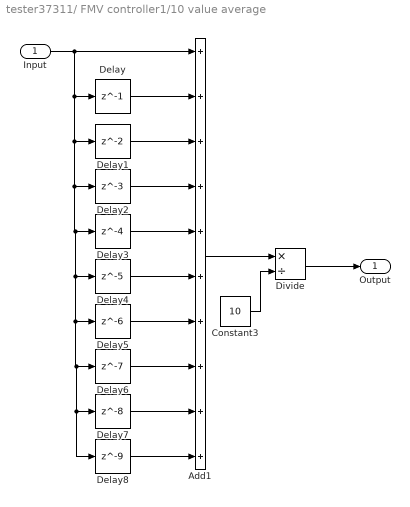
== system tester37311/ FMV controller1/10 value average ==
  Input : Inport
  Add1 : Sum  Inputs=++++++++++
  Constant3 : Constant  Value=10
  Delay : Delay  DelayLength=1  InitialCondition=optimal_rotation
  Delay1 : Delay  InitialCondition=optimal_rotation
  Delay2 : Delay  DelayLength=3  InitialCondition=optimal_rotation
  Delay3 : Delay  DelayLength=4  InitialCondition=optimal_rotation
  Delay4 : Delay  DelayLength=5  InitialCondition=optimal_rotation
  Delay5 : Delay  DelayLength=6  InitialCondition=optimal_rotation
  Delay6 : Delay  DelayLength=7  InitialCondition=optimal_rotation
  Delay7 : Delay  DelayLength=8  InitialCondition=optimal_rotation
  Delay8 : Delay  DelayLength=9  InitialCondition=optimal_rotation
  Divide : Product  Inputs=*/
  Output : Outport
  wires:
  Input/1 -> Delay8/1, Delay7/1, Delay6/1, Delay5/1, Delay4/1, Delay3/1, Delay2/1, Delay1/1, Delay/1, Add1/1
  Delay8/1 -> Add1/10
  Delay2/1 -> Add1/4
  Constant3/1 -> Divide/2
  Add1/1 -> Divide/1
  Divide/1 -> Output/1
  Delay7/1 -> Add1/9
  Delay3/1 -> Add1/5
  Delay6/1 -> Add1/8
  Delay5/1 -> Add1/7
  Delay4/1 -> Add1/6
  Delay/1 -> Add1/2
  Delay1/1 -> Add1/3

== system tester37311/Ng speed limiters/Safe switch ==
  In1 : Inport
  Add1 : Sum
  Delay : Delay  DelayLength=1
  OFF : Constant  Value=0
  ON : Constant
  Switch1 : Switch  Criteria=u2 > Threshold  Threshold=10  SaturateOnIntegerOverflow=off  InputSameDT=off
  min 0 : Saturate  UpperLimit=100  LowerLimit=0
  Out1 : Outport
  wires:
  ON/1 -> Switch1/1
  Delay/1 -> Add1/2
  Add1/1 -> min 0/1
  Switch1/1 -> Out1/1
  min 0/1 -> Switch1/2, Delay/1
  OFF/1 -> Switch1/3
  In1/1 -> Add1/1

== system tester37311/Np speed limiters/Safe switch ==
  In1 : Inport
  Add1 : Sum
  Delay : Delay  DelayLength=1
  OFF : Constant  Value=0
  ON : Constant
  Switch1 : Switch  Criteria=u2 > Threshold  Threshold=10  SaturateOnIntegerOverflow=off  InputSameDT=off
  min 0 : Saturate  UpperLimit=100  LowerLimit=0
  Np to SOV : Outport
  wires:
  ON/1 -> Switch1/1
  Delay/1 -> Add1/2
  Add1/1 -> min 0/1
  Switch1/1 -> Np to SOV/1
  min 0/1 -> Switch1/2, Delay/1
  OFF/1 -> Switch1/3
  In1/1 -> Add1/1

== system tester37311/P3t//P2t limiter/Safe switch ==
  In1 : Inport
  Add1 : Sum
  Delay : Delay  DelayLength=1
  OFF : Constant  Value=0
  ON : Constant
  Switch1 : Switch  Criteria=u2 > Threshold  Threshold=10  SaturateOnIntegerOverflow=off  InputSameDT=off
  min 0 : Saturate  UpperLimit=100  LowerLimit=0
  P3t/P2t to ABV : Outport
  wires:
  ON/1 -> Switch1/1
  Delay/1 -> Add1/2
  Add1/1 -> min 0/1
  Switch1/1 -> P3t/P2t to ABV/1
  min 0/1 -> Switch1/2, Delay/1
  OFF/1 -> Switch1/3
  In1/1 -> Add1/1

== system tester37311/T45t limiter/Safe switch ==
  In1 : Inport
  Add1 : Sum
  Delay : Delay  DelayLength=1
  OFF : Constant  Value=0
  ON : Constant
  Switch1 : Switch  Criteria=u2 > Threshold  Threshold=10  SaturateOnIntegerOverflow=off  InputSameDT=off
  min 0 : Saturate  UpperLimit=100  LowerLimit=0
  T45t to SOV : Outport
  wires:
  ON/1 -> Switch1/1
  Delay/1 -> Add1/2
  Add1/1 -> min 0/1
  Switch1/1 -> T45t to SOV/1
  min 0/1 -> Switch1/2, Delay/1
  OFF/1 -> Switch1/3
  In1/1 -> Add1/1

== system tester37311/Torque limiters/Safe switch ==
  In1 : Inport
  Add1 : Sum
  Delay : Delay  DelayLength=1
  OFF : Constant  Value=0
  ON : Constant
  Switch1 : Switch  Criteria=u2 > Threshold  Threshold=10  SaturateOnIntegerOverflow=off  InputSameDT=off
  min 0 : Saturate  UpperLimit=100  LowerLimit=0
  Torque to SOV : Outport
  wires:
  ON/1 -> Switch1/1
  Delay/1 -> Add1/2
  Add1/1 -> min 0/1
  Switch1/1 -> Torque to SOV/1
  min 0/1 -> Switch1/2, Delay/1
  OFF/1 -> Switch1/3
  In1/1 -> Add1/1

== matlab function tester37311/ FMV controller1/FMV controller ==
  data: dP3P2 input; dT45 input; y output
function y = fcn(dP3P2,dT45)
    u=max(dP3P2,dT45);
y = u;

== matlab function tester37311/MATLAB Function ==
  data: u input; y output
function y = fcn(u)

y = sort(u);

== matlab function tester37311/T45t limiter/T45 VOTER ==
  data: u input; y output
function y = fcn(u)
u=sort(u);
y = (u(2)+u(3)+u(4))/3;
